simulink model "MotorControl"  (R2018b)
settings: Solver=FixedStepDiscrete  StartTime=0.0  StopTime=10.0  FixedStep=sampleTime  RelTol=1e-3  EnableMultiTasking=on
values from neighbouring files (symbols this model uses):
  gearRatio = 3575.0855    [settings.mat]
  sampleTime = 0.01    [settings.mat]
  wheelRadius = 0.02    [settings.mat]
libraries: arduinolib x4, simulink x3
settings Model: ExtModeTrigDuration=2  Creator=KSURCT Officers  LastModifiedBy=Dylan Staatz
settings OptimizationCC: EnhancedBackFolding=on  PassReuseOutputArgsAs=Individual arguments  MaxStackSize=64  OptimizeBlockOrder=speed  DifferentSizesBufferReuse=on  OptimizationCustomize=off
settings DebuggingCC: ParameterTunabilityLossMsg=error
settings HardwareCC: ProdBitPerPointer=32  ProdBitPerSizeT=32  ProdBitPerPtrDiffT=32  ProdLargestAtomicInteger=Long  ProdLargestAtomicFloat=Double  ProdWordSize=32  ProdHWDeviceType=ARM Compatible->ARM Cortex
settings SFSimCC: SimCustomInitializer=analogWriteResolution(12);  MATLABDynamicMemAlloc=off
settings RTWCC: SystemTargetFile=ert.tlc  HardwareBoard=Arduino Due  TemplateMakefile=ert_default_tmf  GenerateReport=on  Toolchain=Arduino ARM  BuildConfiguration=Faster Runs  IncludeHyperlinkInReport=on  LaunchReport=on  GenerateTraceInfo=on  GenerateTraceReport=on  GenerateTraceReportSl=on  GenerateTraceReportSf=on  GenerateTraceReportEml=on
settings CodeAppCC: ForceParamTrailComments=on  IgnoreCustomStorageClasses=off  OperatorAnnotations=on  SimulinkDataObjDesc=on  SFDataObjDesc=on  InsertBlockDesc=on
settings ERTTargetCC: SupportContinuousTime=on  SupportVariableSizeSignals=on

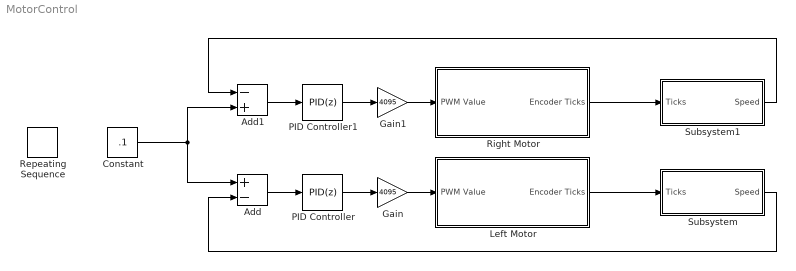
== system MotorControl ==
  Add : Sum  Inputs=+-
  Add1 : Sum  Inputs=-+
  Constant : Constant  Value=.1
  Gain : Gain  Gain=4095
  Gain1 : Gain  Gain=4095
  Left Motor : Subsystem
  PID Controller : simulink/Continuous/PID Controller  Controller=PID  Form=Parallel  TimeDomain=Discrete-time  SampleTime=-1  IntegratorMethod=Forward Euler  FilterMethod=Forward Euler  ControllerParametersSource=internal  P=1e10  I=1e8  D=0  UseFilter=on  N=100  TunerSelectOption=Transfer Function Based (PID Tuner App)  InitialConditionSource=internal  InitialConditionForIntegrator=0  InitialConditionForFilter=0  DifferentiatorICPrevScaledInput=0  ExternalReset=none  TrackingMode=off  Kt=1  LimitOutput=on  UpperSaturationLimit=1  LowerSaturationLimit=-1  LinearizeAsGain=on  AntiWindupMode=none  Kb=1  POutMin=[]  POutMax=[]  IOutMin=[]  IOutMax=[]  DOutMin=[]  DOutMax=[]  NOutMin=[]  NOutMax=[]  SumOutMin=[]  SumOutMax=[]  SaturationOutMin=[]  SaturationOutMax=[]  PParamMin=[]  PParamMax=[]  IParamMin=[]  IParamMax=[]  DParamMin=[]  DParamMax=[]  NParamMin=[]  NParamMax=[]  KbParamMin=[]  KbParamMax=[]  KtParamMin=[]  KtParamMax=[]  KbOutMin=[]  KbOutMax=[]  KtOutMin=[]  KtOutMax=[]  IntegratorOutMin=[]  IntegratorOutMax=[]  FilterOutMin=[]  FilterOutMax=[]  SumI1OutMin=[]  SumI1OutMax=[]  SumI2OutMin=[]  SumI2OutMax=[]  SumI3OutMin=[]  SumI3OutMax=[]  SumI4OutMin=[]  SumI4OutMax=[]  SumDOutMin=[]  SumDOutMax=[]  DifferentiatorOutMin=[]  DifferentiatorOutMax=[]  FilterDiffOutCoefMin=[]  FilterDiffOutCoefMax=[]  ReciprocalOutMin=[]  ReciprocalOutMax=[]  SumDenOutMin=[]  SumDenOutMax=[]  SumNumOutMin=[]  SumNumOutMax=[]  DivideOutMin=[]  DivideOutMax=[]  IntegratorContinuousStateAttributes=''  IntegratorStateMustResolveToSignalObject=off  IntegratorRTWStateStorageClass=Auto  FilterContinuousStateAttributes=''  FilterStateMustResolveToSignalObject=off  FilterRTWStateStorageClass=Auto  ParallelPVariant=InternalParameters  IdealPVariant=Disabled  IVariant=InternalParameters  DVariant=InternalParameters  IntegratorVariant=Discrete  SatVariant=Enabled  AWVariant=Passthrough  PCopyVariant=Disabled  TRVariant=Disabled  FdbkBlocksVariant=Forward  IdealPFdbkVariant=Disabled  SatFdbkVariant=Disabled  DerivativeFilterVariant=ForwardEulerFilter  NVariant=InternalParameters  NCopyVariant=Disabled  FilterICVariant=InternalICsFilter  IntegratorICVariant=InternalICs  ExternalResetVariant=Disabled  TRSumVariant=Passthrough  SumFdbkVariant=Disabled  SumVariant=Sum_PID
  PID Controller1 : simulink/Continuous/PID Controller  Controller=PID  Form=Parallel  TimeDomain=Discrete-time  SampleTime=-1  IntegratorMethod=Forward Euler  FilterMethod=Forward Euler  ControllerParametersSource=internal  P=1e10  I=1e8  D=0  UseFilter=on  N=100  TunerSelectOption=Transfer Function Based (PID Tuner App)  InitialConditionSource=internal  InitialConditionForIntegrator=0  InitialConditionForFilter=0  DifferentiatorICPrevScaledInput=0  ExternalReset=none  TrackingMode=off  Kt=1  LimitOutput=on  UpperSaturationLimit=1  LowerSaturationLimit=-1  LinearizeAsGain=on  AntiWindupMode=none  Kb=1  POutMin=[]  POutMax=[]  IOutMin=[]  IOutMax=[]  DOutMin=[]  DOutMax=[]  NOutMin=[]  NOutMax=[]  SumOutMin=[]  SumOutMax=[]  SaturationOutMin=[]  SaturationOutMax=[]  PParamMin=[]  PParamMax=[]  IParamMin=[]  IParamMax=[]  DParamMin=[]  DParamMax=[]  NParamMin=[]  NParamMax=[]  KbParamMin=[]  KbParamMax=[]  KtParamMin=[]  KtParamMax=[]  KbOutMin=[]  KbOutMax=[]  KtOutMin=[]  KtOutMax=[]  IntegratorOutMin=[]  IntegratorOutMax=[]  FilterOutMin=[]  FilterOutMax=[]  SumI1OutMin=[]  SumI1OutMax=[]  SumI2OutMin=[]  SumI2OutMax=[]  SumI3OutMin=[]  SumI3OutMax=[]  SumI4OutMin=[]  SumI4OutMax=[]  SumDOutMin=[]  SumDOutMax=[]  DifferentiatorOutMin=[]  DifferentiatorOutMax=[]  FilterDiffOutCoefMin=[]  FilterDiffOutCoefMax=[]  ReciprocalOutMin=[]  ReciprocalOutMax=[]  SumDenOutMin=[]  SumDenOutMax=[]  SumNumOutMin=[]  SumNumOutMax=[]  DivideOutMin=[]  DivideOutMax=[]  IntegratorContinuousStateAttributes=''  IntegratorStateMustResolveToSignalObject=off  IntegratorRTWStateStorageClass=Auto  FilterContinuousStateAttributes=''  FilterStateMustResolveToSignalObject=off  FilterRTWStateStorageClass=Auto  ParallelPVariant=InternalParameters  IdealPVariant=Disabled  IVariant=InternalParameters  DVariant=InternalParameters  IntegratorVariant=Discrete  SatVariant=Enabled  AWVariant=Passthrough  PCopyVariant=Disabled  TRVariant=Disabled  FdbkBlocksVariant=Forward  IdealPFdbkVariant=Disabled  SatFdbkVariant=Disabled  DerivativeFilterVariant=ForwardEulerFilter  NVariant=InternalParameters  NCopyVariant=Disabled  FilterICVariant=InternalICsFilter  IntegratorICVariant=InternalICs  ExternalResetVariant=Disabled  TRSumVariant=Passthrough  SumFdbkVariant=Disabled  SumVariant=Sum_PID
  Repeating Sequence : simulink/Sources/Repeating Sequence  rep_seq_t=linspace(0,10, 1000)  rep_seq_y=linspace(-.25,.25, 1000)
  Right Motor : Subsystem
  Subsystem : Subsystem
  Subsystem1 : Subsystem
  wires:
  Add/1 -> PID Controller/1
  PID Controller/1 -> Gain/1
  Gain/1 -> Left Motor/1(PWM Value)
  Left Motor/1(Encoder Ticks) -> Subsystem/1(Ticks)
  Subsystem/1(Speed) -> Add/2
  Subsystem1/1(Speed) -> Add1/1
  Right Motor/1(Encoder Ticks) -> Subsystem1/1(Ticks)
  Gain1/1 -> Right Motor/1(PWM Value)
  PID Controller1/1 -> Gain1/1
  Add1/1 -> PID Controller1/1
  Constant/1 -> Add/1, Add1/2

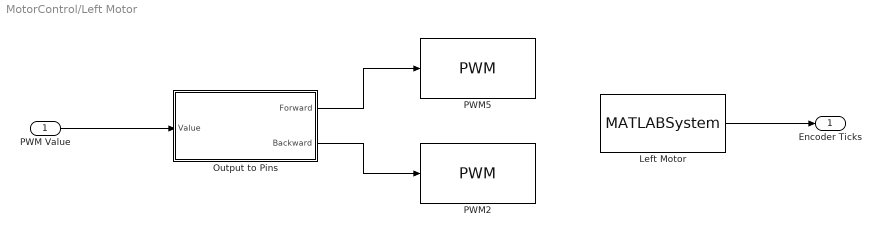
== system MotorControl/Left Motor ==
  PWM Value : Inport
  Left Motor : MATLABSystem  System=EncoderRead  pinA=int8(11)  pinB=int8(10)  id=int8(0)  SampleTime=-1
      mask Type: EncoderRead
      mask Display:
      | disp('Source');
      | port_label('output',1,'ticks');
  Output to Pins : Subsystem
  PWM2 : arduinolib/PWM  pinNumber=2  EnableInputFrequency=off  InitialFrequency=2000  InitialDutyCycle=0  NotificationType=None  blockPlatform=arduino
  PWM5 : arduinolib/PWM  pinNumber=3  EnableInputFrequency=off  InitialFrequency=2000  InitialDutyCycle=0  NotificationType=None  blockPlatform=arduino
  Encoder Ticks : Outport
  wires:
  Output to Pins/2("Backward ") -> PWM2/1
  Output to Pins/1(Forward) -> PWM5/1
  PWM Value/1 -> Output to Pins/1(Value)
  Left Motor/1 -> Encoder Ticks/1

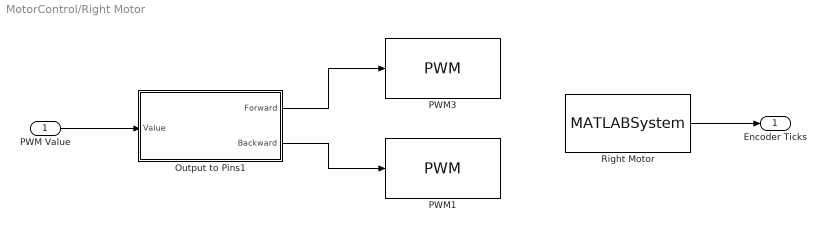
== system MotorControl/Right Motor ==
  PWM Value : Inport
  Output to Pins1 : Subsystem
  PWM1 : arduinolib/PWM  pinNumber=4  EnableInputFrequency=off  InitialFrequency=2000  InitialDutyCycle=0  NotificationType=None  blockPlatform=arduino
  PWM3 : arduinolib/PWM  pinNumber=5  EnableInputFrequency=off  InitialFrequency=2000  InitialDutyCycle=0  NotificationType=None  blockPlatform=arduino
  Right Motor : MATLABSystem  System=EncoderRead  pinA=int8(13)  pinB=int8(12)  id=int8(1)  SampleTime=-1
      mask Type: EncoderRead
      mask Display:
      | disp('Source');
      | port_label('output',1,'ticks');
  Encoder Ticks : Outport
  wires:
  Output to Pins1/2("Backward ") -> PWM1/1
  PWM Value/1 -> Output to Pins1/1(Value)
  Output to Pins1/1(Forward) -> PWM3/1
  Right Motor/1 -> Encoder Ticks/1

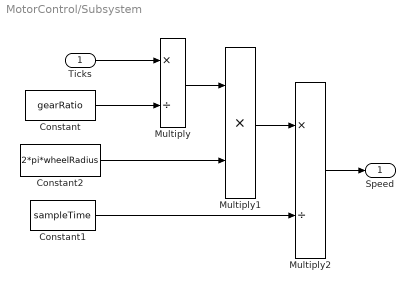
== system MotorControl/Subsystem ==
  Ticks : Inport
  Constant : Constant  Value=gearRatio
  Constant1 : Constant  Value=sampleTime
  Constant2 : Constant  Value=2*pi*wheelRadius
  Multiply : Product  Inputs=*/
  Multiply1 : Product  Inputs=**
  Multiply2 : Product  Inputs=*/
  Speed : Outport
  wires:
  Ticks/1 -> Multiply/1
  Constant/1 -> Multiply/2
  Constant2/1 -> Multiply1/2
  Multiply/1 -> Multiply1/1
  Constant1/1 -> Multiply2/2
  Multiply1/1 -> Multiply2/1
  Multiply2/1 -> Speed/1

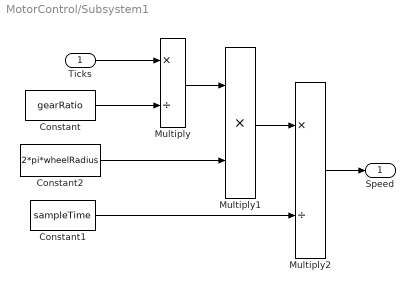
== system MotorControl/Subsystem1 ==
  Ticks : Inport
  Constant : Constant  Value=gearRatio
  Constant1 : Constant  Value=sampleTime
  Constant2 : Constant  Value=2*pi*wheelRadius
  Multiply : Product  Inputs=*/
  Multiply1 : Product  Inputs=**
  Multiply2 : Product  Inputs=*/
  Speed : Outport
  wires:
  Multiply2/1 -> Speed/1
  Multiply1/1 -> Multiply2/1
  Constant1/1 -> Multiply2/2
  Multiply/1 -> Multiply1/1
  Constant2/1 -> Multiply1/2
  Constant/1 -> Multiply/2
  Ticks/1 -> Multiply/1

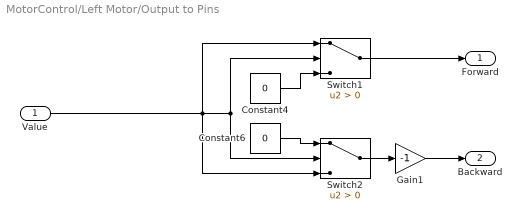
== system MotorControl/Left Motor/Output to Pins ==
  Value : Inport
  Constant4 : Constant  Value=0
  Constant6 : Constant  Value=0
  Gain1 : Gain  Gain=-1
  Switch1 : Switch  Criteria=u2 > Threshold
  Switch2 : Switch  Criteria=u2 > Threshold
  Forward : Outport
  "Backward " : Outport  Port=2
  wires:
  Value/1 -> Switch2/2, Switch1/2, Switch2/3, Switch1/1
  Constant4/1 -> Switch1/3
  Gain1/1 -> "Backward "/1
  Switch2/1 -> Gain1/1
  Constant6/1 -> Switch2/1
  Switch1/1 -> Forward/1

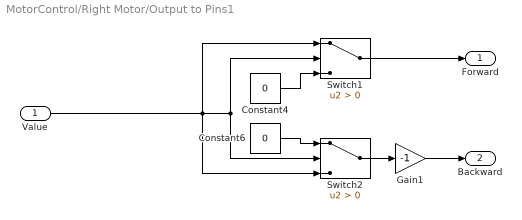
== system MotorControl/Right Motor/Output to Pins1 ==
  Value : Inport
  Constant4 : Constant  Value=0
  Constant6 : Constant  Value=0
  Gain1 : Gain  Gain=-1
  Switch1 : Switch  Criteria=u2 > Threshold
  Switch2 : Switch  Criteria=u2 > Threshold
  Forward : Outport
  "Backward " : Outport  Port=2
  wires:
  Switch1/1 -> Forward/1
  Constant6/1 -> Switch2/1
  Switch2/1 -> Gain1/1
  Gain1/1 -> "Backward "/1
  Constant4/1 -> Switch1/3
  Value/1 -> Switch1/1, Switch2/3, Switch1/2, Switch2/2
